simulink model "colorDetectionPID"  (R2022b)
settings: Solver=ode1  StartTime=0.0  StopTime=inf  FixedStep=0.001  RelTol=1e-9
model workspace (MAT data in the model file):
  SL_ROS_VariableLengthArrays_MaxSizes.CommonInfo.ArrayTruncateAction = 'EmitWarning'
  SL_ROS_VariableLengthArrays_MaxSizes.MsgTypeMap = containers.Map
  SL_ROS_VariableLengthArrays_MaxSizes.MsgTypeMap.serialization.keys = {'sensor_msgs/CompressedImage'}
  SL_ROS_VariableLengthArrays_MaxSizes.MsgTypeMap.serialization.values{1}(1).PropertyName = 'Data'
  SL_ROS_VariableLengthArrays_MaxSizes.MsgTypeMap.serialization.values{1}(1).DataType = 'uint8'
  SL_ROS_VariableLengthArrays_MaxSizes.MsgTypeMap.serialization.values{1}(1).MaxLength = 300000
  SL_ROS_VariableLengthArrays_MaxSizes.MsgTypeMap.serialization.values{1}(2).PropertyName = 'Format'
  SL_ROS_VariableLengthArrays_MaxSizes.MsgTypeMap.serialization.values{1}(2).DataType = 'uint8'
  SL_ROS_VariableLengthArrays_MaxSizes.MsgTypeMap.serialization.values{1}(2).MaxLength = 128
  SL_ROS_VariableLengthArrays_MaxSizes.MsgTypeMap.serialization.uniformity = 0
  SL_ROS_VariableLengthArrays_MaxSizes.MsgTypeMap.serialization.keyType = 'char'
  SL_ROS_VariableLengthArrays_MaxSizes.MsgTypeMap.serialization.valueType = 'any'
undefined symbols (not defined in the file): gray, VelLeft, VelRight
libraries: robotlib x11, slpidlib x5, simulink_extras x2, visionsinks x1
settings Model: Creator=domen  LastModifiedBy=gaetano
settings OptimizationCC: EnhancedBackFolding=on  PassReuseOutputArgsAs=Individual arguments  ZeroExternalMemoryAtStartup=off  ZeroInternalMemoryAtStartup=off  MaxStackSize=64  OptimizeBlockOrder=speed  DifferentSizesBufferReuse=on  OptimizationCustomize=off  EfficientTunableParamExpr=on
settings DebuggingCC: ParameterTunabilityLossMsg=error
settings HardwareCC: ProdBitPerPointer=32  ProdBitPerSizeT=32  ProdBitPerPtrDiffT=32  ProdLargestAtomicFloat=None  ProdIntDivRoundTo=Undefined  ProdEndianess=Unspecified  ProdWordSize=32  ProdHWDeviceType=Generic->Unspecified (assume 32-bit Generic)  UseEmbeddedCoderFeatures=off
settings RTWCC: Description=Embedded Coder  SystemTargetFile=ert.tlc  HardwareBoard=Robot Operating System (ROS)  TLCOptions="-aInlineSetEventsForThisBaseRateFcn=TLC_FALSE -aSuppressMultiTaskScheduler=TLC_FALSE  -aRateBasedStepFcn=0"  TemplateMakefile=ert_default_tmf  Toolchain=Catkin  TargetLang=C++
settings CodeAppCC: ForceParamTrailComments=on  IgnoreCustomStorageClasses=off  OperatorAnnotations=on  SimulinkDataObjDesc=on  SFDataObjDesc=on  InsertBlockDesc=on
settings ERTTargetCC: SupportNonInlinedSFcns=on

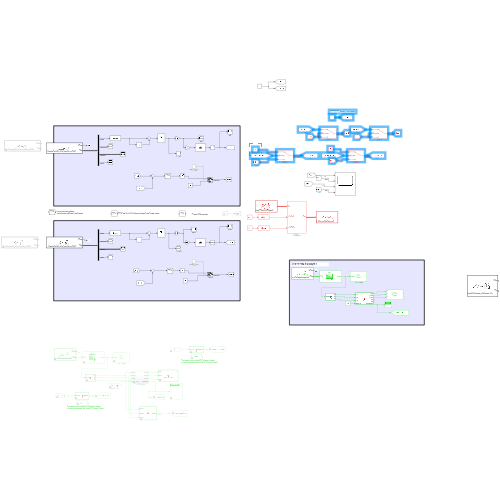
[thumbnail: Simulink's stored preview of the top-level diagram]
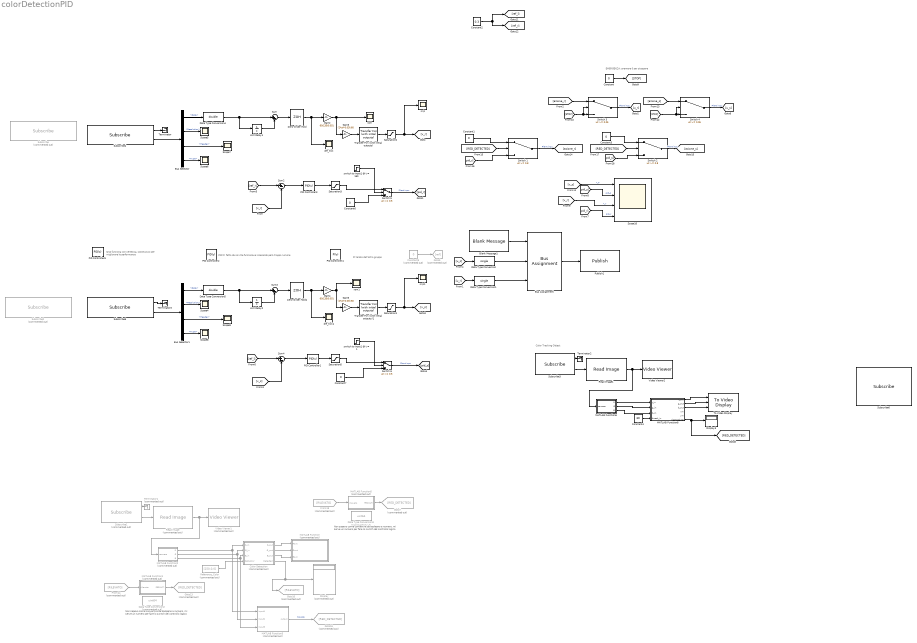
== system colorDetectionPID ==
  note: Color Tracking Object
  note: Non sapevo come convertire da booleano a numero,
      | mi serve un numero per fare lo switch del controllo logico
  note: EMERGENZA: premere 0 per stoppare
  note: 6/12 funziona con certezza,
      |  sostituisco per migliorare le performance
  note: PID(z) fatto da noi che funzionava inserendo però troppo rumore
  note: PI tarato dall'altro gruppo
  note: Non sapevo come convertire da booleano a numero,
      | mi serve un numero per fare lo switch del controllo logico
  Blank Message1 : robotlib/Blank Message  messageClass=Message  entityType=duckietown_msgs/WheelsCmdStamped  messageType=duckietown_msgs/WheelsCmdStamped  SampleTime=-1  legacyBusStruct=off
      settings: LibrarySourceBlock=roslib/ROS/Blank Message
  Bus Assignment : BusAssignment  AssignedSignals=VelLeft,VelRight
  Bus Selector : BusSelector  OutputSignals=Data,Resolution,Header,Type
  Bus Selector1 : BusSelector  OutputSignals=Data,Resolution,Header,Type
  Color Detection : Subsystem  Commented=on
  Constant{,1,3,6..7} (5 alike) : Constant  Value=0
  Constant2 : Constant  Value=0.3
  Constant4 : Constant  Value=30
  Constant5 : Constant  Commented=on  Value=0
  Data Type Conversion : DataTypeConversion  OutDataTypeStr=single  SaturateOnIntegerOverflow=off  RndMeth=Floor
  Data Type Conversion1 : DataTypeConversion  OutDataTypeStr=single  SaturateOnIntegerOverflow=off  RndMeth=Floor
  Data Type Conversion2 : DataTypeConversion  Commented=on  OutMin=[0]  OutMax=[1]  OutDataTypeStr=uint64  SaturateOnIntegerOverflow=off  RndMeth=Floor
  Data Type Conversion3 : DataTypeConversion  Commented=on  OutMin=[0]  OutMax=[1]  OutDataTypeStr=uint64  SaturateOnIntegerOverflow=off  RndMeth=Floor
  Data Type Conversion4 : DataTypeConversion  OutDataTypeStr=double  SaturateOnIntegerOverflow=off  RndMeth=Floor
  Data Type Conversion5 : DataTypeConversion  OutDataTypeStr=double  SaturateOnIntegerOverflow=off  RndMeth=Floor
  Display : Display  Commented=on
  Display3 : Display
  From14 : From  Commented=on  GotoTag=RILEVATO
  From19 : From  Commented=on  GotoTag=RILEVATO
  Gain2 : Gain  Gain=60/135/0.001
  Gain3 : Gain  Gain=(2*pi*0.03)/60
  Gain4 : Gain  Gain=60/135/0.001
  Gain5 : Gain  Gain=(2*pi*0.03)/60
  Goto10 : Goto  Commented=on  GotoTag=RILEVATO
  Goto13 : Goto  Commented=on  GotoTag=RED_DETECTED
  Goto16 : Goto  Commented=on  GotoTag=RED_DETECTED
  Goto5 : Goto  Commented=on  GotoTag=ref
  Goto7 : Goto  Commented=on  GotoTag=RED_DETECTED
  MATLAB Function : MATLAB Function  Commented=on  TreatAsAtomicUnit=on
  MATLAB Function1 : MATLAB Function  Commented=on  TreatAsAtomicUnit=on
  MATLAB Function2 : MATLAB Function  Commented=on  TreatAsAtomicUnit=on
  MATLAB Function3 : MATLAB Function  Commented=on  TreatAsAtomicUnit=on
  MATLAB Function5 : MATLAB Function  Commented=on  TreatAsAtomicUnit=on
  MATLAB Function6 : MATLAB Function  TreatAsAtomicUnit=on
  MATLAB Function8 : MATLAB Function  TreatAsAtomicUnit=on
  PID Controller1 : slpidlib/PID Controller  Controller=PID  Form=Parallel  TimeDomain=Continuous-time  UseExternalTs=off  SampleTime=-1  IntegratorMethod=Forward Euler  FilterMethod=Forward Euler  ControllerParametersSource=internal  P=1.339  I=1.386  UseKiTs=off  D=0.111  N=2.50192573013059  UseFilter=on  TunerSelectOption=Transfer Function Based (PID Tuner App)  InitialConditionSource=internal  InitialConditionForIntegrator=0  InitialConditionForFilter=0  DifferentiatorICPrevScaledInput=0  ExternalReset=none  TrackingMode=off  Kt=1  LimitOutput=off  SatLimitsSource=internal  UpperSaturationLimit=inf  LowerSaturationLimit=-inf  LinearizeAsGain=on  AntiWindupMode=none  Kb=1  LimitIntegrator=off  UpperIntegratorSaturationLimit=inf  LowerIntegratorSaturationLimit=-inf  POutMin=[]  POutMax=[]  IOutMin=[]  IOutMax=[]  DOutMin=[]  DOutMax=[]  NOutMin=[]  NOutMax=[]  SumOutMin=[]  SumOutMax=[]  SaturationOutMin=[]  SaturationOutMax=[]  PParamMin=[]  PParamMax=[]  IParamMin=[]  IParamMax=[]  DParamMin=[]  DParamMax=[]  NParamMin=[]  NParamMax=[]  KbParamMin=[]  KbParamMax=[]  KtParamMin=[]  KtParamMax=[]  KbOutMin=[]  KbOutMax=[]  KtOutMin=[]  KtOutMax=[]  IntegratorOutMin=[]  IntegratorOutMax=[]  FilterOutMin=[]  FilterOutMax=[]  SumI1OutMin=[]  SumI1OutMax=[]  SumI2OutMin=[]  SumI2OutMax=[]  SumI3OutMin=[]  SumI3OutMax=[]  SumI4OutMin=[]  SumI4OutMax=[]  SumDOutMin=[]  SumDOutMax=[]  DifferentiatorOutMin=[]  DifferentiatorOutMax=[]  FilterDiffOutCoefMin=[]  FilterDiffOutCoefMax=[]  ReciprocalOutMin=[]  ReciprocalOutMax=[]  SumDenOutMin=[]  SumDenOutMax=[]  SumNumOutMin=[]  SumNumOutMax=[]  DivideOutMin=[]  DivideOutMax=[]  UdiffTsProdOutMin=[]  UdiffTsProdOutMax=[]  NTsProdOutMin=[]  NTsProdOutMax=[]  UintegralTsProdOutMin=[]  UintegralTsProdOutMax=[]  UngainTsProdOutMin=[]  UngainTsProdOutMax=[]  ClampingZeroOutDataTypeStr=Inherit: Inherit via back propagation  ClampingZeroOutMin=[]  ClampingZeroOutMax=[]  FilterDenConstantOutDataTypeStr=Inherit: Inherit via back propagation  FilterDenConstantOutMin=[]  FilterDenConstantOutMax=[]  PCopyOutDataTypeStr=Inherit: Inherit via back propagation  PCopyOutMin=[]  PCopyOutMax=[]  NCopyOutDataTypeStr=Inherit: Inherit via back propagation  NCopyOutMin=[]  NCopyOutMax=[]  IntegratorContinuousStateAttributes=''  IntegratorStateMustResolveToSignalObject=off  IntegratorRTWStateStorageClass=Auto  FilterContinuousStateAttributes=''  FilterStateMustResolveToSignalObject=off  FilterRTWStateStorageClass=Auto  ParallelPVariant=InternalParameters  IdealPVariant=Disabled  IVariant=InternalParameters  DVariant=InternalParameters  IntegratorVariant=Continuous  SatVariant=Disabled  AWVariant=Passthrough  PCopyVariant=Disabled  TRVariant=Disabled  FdbkBlocksVariant=Forward  IdealPFdbkVariant=Disabled  SatFdbkVariant=Disabled  DerivativeFilterVariant=ContFilter  NVariant=InternalParameters  NCopyVariant=Disabled  FilterICVariant=InternalICsFilter  IntegratorICVariant=InternalICs  ExternalResetVariant=Disabled  TRSumVariant=Passthrough  SumFdbkVariant=Disabled  SumVariant=Sum_PID  TsampFilterVariant=InternalTs  TsampNgainVariant=Passthrough  TsampIntegralVariant=Passthrough  ExternalSaturationOutDataTypeStr=Inherit: Same as second input
  PID Controller2 : slpidlib/PID Controller  Controller=PID  Form=Parallel  TimeDomain=Discrete-time  UseExternalTs=off  SampleTime=-1  IntegratorMethod=Forward Euler  FilterMethod=Forward Euler  ControllerParametersSource=internal  P=1.9258578338098  I=1.64428587710628  UseKiTs=off  D=0.231536267148539  N=3.35803573669718  UseFilter=on  TunerSelectOption=Transfer Function Based (PID Tuner App)  InitialConditionSource=internal  InitialConditionForIntegrator=0  InitialConditionForFilter=0  DifferentiatorICPrevScaledInput=0  ExternalReset=none  TrackingMode=off  Kt=1  LimitOutput=off  SatLimitsSource=internal  UpperSaturationLimit=inf  LowerSaturationLimit=-inf  LinearizeAsGain=on  AntiWindupMode=none  Kb=1  LimitIntegrator=off  UpperIntegratorSaturationLimit=inf  LowerIntegratorSaturationLimit=-inf  POutMin=[]  POutMax=[]  IOutMin=[]  IOutMax=[]  DOutMin=[]  DOutMax=[]  NOutMin=[]  NOutMax=[]  SumOutMin=[]  SumOutMax=[]  SaturationOutMin=[]  SaturationOutMax=[]  PParamMin=[]  PParamMax=[]  IParamMin=[]  IParamMax=[]  DParamMin=[]  DParamMax=[]  NParamMin=[]  NParamMax=[]  KbParamMin=[]  KbParamMax=[]  KtParamMin=[]  KtParamMax=[]  KbOutMin=[]  KbOutMax=[]  KtOutMin=[]  KtOutMax=[]  IntegratorOutMin=[]  IntegratorOutMax=[]  FilterOutMin=[]  FilterOutMax=[]  SumI1OutMin=[]  SumI1OutMax=[]  SumI2OutMin=[]  SumI2OutMax=[]  SumI3OutMin=[]  SumI3OutMax=[]  SumI4OutMin=[]  SumI4OutMax=[]  SumDOutMin=[]  SumDOutMax=[]  DifferentiatorOutMin=[]  DifferentiatorOutMax=[]  FilterDiffOutCoefMin=[]  FilterDiffOutCoefMax=[]  ReciprocalOutMin=[]  ReciprocalOutMax=[]  SumDenOutMin=[]  SumDenOutMax=[]  SumNumOutMin=[]  SumNumOutMax=[]  DivideOutMin=[]  DivideOutMax=[]  UdiffTsProdOutMin=[]  UdiffTsProdOutMax=[]  NTsProdOutMin=[]  NTsProdOutMax=[]  UintegralTsProdOutMin=[]  UintegralTsProdOutMax=[]  UngainTsProdOutMin=[]  UngainTsProdOutMax=[]  ClampingZeroOutDataTypeStr=Inherit: Inherit via back propagation  ClampingZeroOutMin=[]  ClampingZeroOutMax=[]  FilterDenConstantOutDataTypeStr=Inherit: Inherit via back propagation  FilterDenConstantOutMin=[]  FilterDenConstantOutMax=[]  PCopyOutDataTypeStr=Inherit: Inherit via back propagation  PCopyOutMin=[]  PCopyOutMax=[]  NCopyOutDataTypeStr=Inherit: Inherit via back propagation  NCopyOutMin=[]  NCopyOutMax=[]  IntegratorContinuousStateAttributes=''  IntegratorStateMustResolveToSignalObject=off  IntegratorRTWStateStorageClass=Auto  FilterContinuousStateAttributes=''  FilterStateMustResolveToSignalObject=off  FilterRTWStateStorageClass=Auto  ParallelPVariant=InternalParameters  IdealPVariant=Disabled  IVariant=InternalParameters  DVariant=InternalParameters  IntegratorVariant=Discrete  SatVariant=Disabled  AWVariant=Passthrough  PCopyVariant=Disabled  TRVariant=Disabled  FdbkBlocksVariant=Forward  IdealPFdbkVariant=Disabled  SatFdbkVariant=Disabled  DerivativeFilterVariant=ForwardEulerFilter  NVariant=InternalParameters  NCopyVariant=Disabled  FilterICVariant=InternalICsFilter  IntegratorICVariant=InternalICs  ExternalResetVariant=Disabled  TRSumVariant=Passthrough  SumFdbkVariant=Disabled  SumVariant=Sum_PID  TsampFilterVariant=InternalTs  TsampNgainVariant=Passthrough  TsampIntegralVariant=Passthrough  ExternalSaturationOutDataTypeStr=Inherit: Same as second input
  PID Controller3 : slpidlib/PID Controller  Controller=PID  Form=Parallel  TimeDomain=Continuous-time  UseExternalTs=off  SampleTime=-1  IntegratorMethod=Forward Euler  FilterMethod=Forward Euler  ControllerParametersSource=internal  P=1.339  I=1.386  UseKiTs=off  D=0.111  N=2.50192573013059  UseFilter=on  TunerSelectOption=Transfer Function Based (PID Tuner App)  InitialConditionSource=internal  InitialConditionForIntegrator=0  InitialConditionForFilter=0  DifferentiatorICPrevScaledInput=0  ExternalReset=none  TrackingMode=off  Kt=1  LimitOutput=off  SatLimitsSource=internal  UpperSaturationLimit=inf  LowerSaturationLimit=-inf  LinearizeAsGain=on  AntiWindupMode=none  Kb=1  LimitIntegrator=off  UpperIntegratorSaturationLimit=inf  LowerIntegratorSaturationLimit=-inf  POutMin=[]  POutMax=[]  IOutMin=[]  IOutMax=[]  DOutMin=[]  DOutMax=[]  NOutMin=[]  NOutMax=[]  SumOutMin=[]  SumOutMax=[]  SaturationOutMin=[]  SaturationOutMax=[]  PParamMin=[]  PParamMax=[]  IParamMin=[]  IParamMax=[]  DParamMin=[]  DParamMax=[]  NParamMin=[]  NParamMax=[]  KbParamMin=[]  KbParamMax=[]  KtParamMin=[]  KtParamMax=[]  KbOutMin=[]  KbOutMax=[]  KtOutMin=[]  KtOutMax=[]  IntegratorOutMin=[]  IntegratorOutMax=[]  FilterOutMin=[]  FilterOutMax=[]  SumI1OutMin=[]  SumI1OutMax=[]  SumI2OutMin=[]  SumI2OutMax=[]  SumI3OutMin=[]  SumI3OutMax=[]  SumI4OutMin=[]  SumI4OutMax=[]  SumDOutMin=[]  SumDOutMax=[]  DifferentiatorOutMin=[]  DifferentiatorOutMax=[]  FilterDiffOutCoefMin=[]  FilterDiffOutCoefMax=[]  ReciprocalOutMin=[]  ReciprocalOutMax=[]  SumDenOutMin=[]  SumDenOutMax=[]  SumNumOutMin=[]  SumNumOutMax=[]  DivideOutMin=[]  DivideOutMax=[]  UdiffTsProdOutMin=[]  UdiffTsProdOutMax=[]  NTsProdOutMin=[]  NTsProdOutMax=[]  UintegralTsProdOutMin=[]  UintegralTsProdOutMax=[]  UngainTsProdOutMin=[]  UngainTsProdOutMax=[]  ClampingZeroOutDataTypeStr=Inherit: Inherit via back propagation  ClampingZeroOutMin=[]  ClampingZeroOutMax=[]  FilterDenConstantOutDataTypeStr=Inherit: Inherit via back propagation  FilterDenConstantOutMin=[]  FilterDenConstantOutMax=[]  PCopyOutDataTypeStr=Inherit: Inherit via back propagation  PCopyOutMin=[]  PCopyOutMax=[]  NCopyOutDataTypeStr=Inherit: Inherit via back propagation  NCopyOutMin=[]  NCopyOutMax=[]  IntegratorContinuousStateAttributes=''  IntegratorStateMustResolveToSignalObject=off  IntegratorRTWStateStorageClass=Auto  FilterContinuousStateAttributes=''  FilterStateMustResolveToSignalObject=off  FilterRTWStateStorageClass=Auto  ParallelPVariant=InternalParameters  IdealPVariant=Disabled  IVariant=InternalParameters  DVariant=InternalParameters  IntegratorVariant=Continuous  SatVariant=Disabled  AWVariant=Passthrough  PCopyVariant=Disabled  TRVariant=Disabled  FdbkBlocksVariant=Forward  IdealPFdbkVariant=Disabled  SatFdbkVariant=Disabled  DerivativeFilterVariant=ContFilter  NVariant=InternalParameters  NCopyVariant=Disabled  FilterICVariant=InternalICsFilter  IntegratorICVariant=InternalICs  ExternalResetVariant=Disabled  TRSumVariant=Passthrough  SumFdbkVariant=Disabled  SumVariant=Sum_PID  TsampFilterVariant=InternalTs  TsampNgainVariant=Passthrough  TsampIntegralVariant=Passthrough  ExternalSaturationOutDataTypeStr=Inherit: Same as second input
  PID Controller4 : slpidlib/PID Controller  Controller=PI  Form=Parallel  TimeDomain=Continuous-time  UseExternalTs=off  SampleTime=-1  IntegratorMethod=Forward Euler  FilterMethod=Forward Euler  ControllerParametersSource=internal  P=1  I=0.15  UseKiTs=off  D=0  N=100  UseFilter=on  TunerSelectOption=Transfer Function Based (PID Tuner App)  InitialConditionSource=internal  InitialConditionForIntegrator=0  InitialConditionForFilter=0  DifferentiatorICPrevScaledInput=0  ExternalReset=none  TrackingMode=off  Kt=1  LimitOutput=off  SatLimitsSource=internal  UpperSaturationLimit=inf  LowerSaturationLimit=-inf  LinearizeAsGain=on  AntiWindupMode=none  Kb=1  LimitIntegrator=off  UpperIntegratorSaturationLimit=inf  LowerIntegratorSaturationLimit=-inf  POutMin=[]  POutMax=[]  IOutMin=[]  IOutMax=[]  DOutMin=[]  DOutMax=[]  NOutMin=[]  NOutMax=[]  SumOutMin=[]  SumOutMax=[]  SaturationOutMin=[]  SaturationOutMax=[]  PParamMin=[]  PParamMax=[]  IParamMin=[]  IParamMax=[]  DParamMin=[]  DParamMax=[]  NParamMin=[]  NParamMax=[]  KbParamMin=[]  KbParamMax=[]  KtParamMin=[]  KtParamMax=[]  KbOutMin=[]  KbOutMax=[]  KtOutMin=[]  KtOutMax=[]  IntegratorOutMin=[]  IntegratorOutMax=[]  FilterOutMin=[]  FilterOutMax=[]  SumI1OutMin=[]  SumI1OutMax=[]  SumI2OutMin=[]  SumI2OutMax=[]  SumI3OutMin=[]  SumI3OutMax=[]  SumI4OutMin=[]  SumI4OutMax=[]  SumDOutMin=[]  SumDOutMax=[]  DifferentiatorOutMin=[]  DifferentiatorOutMax=[]  FilterDiffOutCoefMin=[]  FilterDiffOutCoefMax=[]  ReciprocalOutMin=[]  ReciprocalOutMax=[]  SumDenOutMin=[]  SumDenOutMax=[]  SumNumOutMin=[]  SumNumOutMax=[]  DivideOutMin=[]  DivideOutMax=[]  UdiffTsProdOutMin=[]  UdiffTsProdOutMax=[]  NTsProdOutMin=[]  NTsProdOutMax=[]  UintegralTsProdOutMin=[]  UintegralTsProdOutMax=[]  UngainTsProdOutMin=[]  UngainTsProdOutMax=[]  ClampingZeroOutDataTypeStr=Inherit: Inherit via back propagation  ClampingZeroOutMin=[]  ClampingZeroOutMax=[]  FilterDenConstantOutDataTypeStr=Inherit: Inherit via back propagation  FilterDenConstantOutMin=[]  FilterDenConstantOutMax=[]  PCopyOutDataTypeStr=Inherit: Inherit via back propagation  PCopyOutMin=[]  PCopyOutMax=[]  NCopyOutDataTypeStr=Inherit: Inherit via back propagation  NCopyOutMin=[]  NCopyOutMax=[]  IntegratorContinuousStateAttributes=''  IntegratorStateMustResolveToSignalObject=off  IntegratorRTWStateStorageClass=Auto  FilterContinuousStateAttributes=''  FilterStateMustResolveToSignalObject=off  FilterRTWStateStorageClass=Auto  ParallelPVariant=InternalParameters  IdealPVariant=Disabled  IVariant=InternalParameters  DVariant=Disabled  IntegratorVariant=Continuous  SatVariant=Disabled  AWVariant=Passthrough  PCopyVariant=Disabled  TRVariant=Disabled  FdbkBlocksVariant=Forward  IdealPFdbkVariant=Disabled  SatFdbkVariant=Disabled  DerivativeFilterVariant=Disabled  NVariant=Disabled  NCopyVariant=Disabled_SignalSpec  FilterICVariant=Disabled  IntegratorICVariant=InternalICs  ExternalResetVariant=Disabled  TRSumVariant=Passthrough  SumFdbkVariant=Disabled  SumVariant=Sum_PI  TsampFilterVariant=InternalTs  TsampNgainVariant=Passthrough  TsampIntegralVariant=Passthrough  ExternalSaturationOutDataTypeStr=Inherit: Same as second input
  PID Controller6 : slpidlib/PID Controller  Controller=PID  Form=Parallel  TimeDomain=Continuous-time  UseExternalTs=off  SampleTime=-1  IntegratorMethod=Forward Euler  FilterMethod=Forward Euler  ControllerParametersSource=internal  P=1.9500021729767  I=2.64652436503106  UseKiTs=off  D=0.143645278367384  N=3.78681783159113  UseFilter=on  TunerSelectOption=Transfer Function Based (PID Tuner App)  InitialConditionSource=internal  InitialConditionForIntegrator=0  InitialConditionForFilter=0  DifferentiatorICPrevScaledInput=0  ExternalReset=none  TrackingMode=off  Kt=1  LimitOutput=off  SatLimitsSource=internal  UpperSaturationLimit=inf  LowerSaturationLimit=-inf  LinearizeAsGain=on  AntiWindupMode=none  Kb=1  LimitIntegrator=off  UpperIntegratorSaturationLimit=inf  LowerIntegratorSaturationLimit=-inf  POutMin=[]  POutMax=[]  IOutMin=[]  IOutMax=[]  DOutMin=[]  DOutMax=[]  NOutMin=[]  NOutMax=[]  SumOutMin=[]  SumOutMax=[]  SaturationOutMin=[]  SaturationOutMax=[]  PParamMin=[]  PParamMax=[]  IParamMin=[]  IParamMax=[]  DParamMin=[]  DParamMax=[]  NParamMin=[]  NParamMax=[]  KbParamMin=[]  KbParamMax=[]  KtParamMin=[]  KtParamMax=[]  KbOutMin=[]  KbOutMax=[]  KtOutMin=[]  KtOutMax=[]  IntegratorOutMin=[]  IntegratorOutMax=[]  FilterOutMin=[]  FilterOutMax=[]  SumI1OutMin=[]  SumI1OutMax=[]  SumI2OutMin=[]  SumI2OutMax=[]  SumI3OutMin=[]  SumI3OutMax=[]  SumI4OutMin=[]  SumI4OutMax=[]  SumDOutMin=[]  SumDOutMax=[]  DifferentiatorOutMin=[]  DifferentiatorOutMax=[]  FilterDiffOutCoefMin=[]  FilterDiffOutCoefMax=[]  ReciprocalOutMin=[]  ReciprocalOutMax=[]  SumDenOutMin=[]  SumDenOutMax=[]  SumNumOutMin=[]  SumNumOutMax=[]  DivideOutMin=[]  DivideOutMax=[]  UdiffTsProdOutMin=[]  UdiffTsProdOutMax=[]  NTsProdOutMin=[]  NTsProdOutMax=[]  UintegralTsProdOutMin=[]  UintegralTsProdOutMax=[]  UngainTsProdOutMin=[]  UngainTsProdOutMax=[]  ClampingZeroOutDataTypeStr=Inherit: Inherit via back propagation  ClampingZeroOutMin=[]  ClampingZeroOutMax=[]  FilterDenConstantOutDataTypeStr=Inherit: Inherit via back propagation  FilterDenConstantOutMin=[]  FilterDenConstantOutMax=[]  PCopyOutDataTypeStr=Inherit: Inherit via back propagation  PCopyOutMin=[]  PCopyOutMax=[]  NCopyOutDataTypeStr=Inherit: Inherit via back propagation  NCopyOutMin=[]  NCopyOutMax=[]  IntegratorContinuousStateAttributes=''  IntegratorStateMustResolveToSignalObject=off  IntegratorRTWStateStorageClass=Auto  FilterContinuousStateAttributes=''  FilterStateMustResolveToSignalObject=off  FilterRTWStateStorageClass=Auto  ParallelPVariant=InternalParameters  IdealPVariant=Disabled  IVariant=InternalParameters  DVariant=InternalParameters  IntegratorVariant=Continuous  SatVariant=Disabled  AWVariant=Passthrough  PCopyVariant=Disabled  TRVariant=Disabled  FdbkBlocksVariant=Forward  IdealPFdbkVariant=Disabled  SatFdbkVariant=Disabled  DerivativeFilterVariant=ContFilter  NVariant=InternalParameters  NCopyVariant=Disabled  FilterICVariant=InternalICsFilter  IntegratorICVariant=InternalICs  ExternalResetVariant=Disabled  TRSumVariant=Passthrough  SumFdbkVariant=Disabled  SumVariant=Sum_PID  TsampFilterVariant=InternalTs  TsampNgainVariant=Passthrough  TsampIntegralVariant=Passthrough  ExternalSaturationOutDataTypeStr=Inherit: Same as second input
  Publish1 : robotlib/Publish  topicSource=Select from ROS network  topic=/vic9osimhen/wheels_driver_node/wheels_cmd  messageType=duckietown_msgs/WheelsCmdStamped  legacyBusStruct=off  messageQueueLength=1
      settings: LibrarySourceBlock=roslib/ROS/Publish
  Read Image : robotlib/Read Image  Commented=on  MaximumImageSize=[ 2000, 2000 ]  ImageEncoding=rgb8  ShowAlphaOutput=off  ShowErrorCodeOutput=off  VariableSizeOutputs=off
      settings: LibrarySourceBlock=roslib/ROS/Read Image
  Read Image1 : robotlib/Read Image  MaximumImageSize=[480, 640 ]  ImageEncoding=rgb8  ShowAlphaOutput=off  ShowErrorCodeOutput=off  VariableSizeOutputs=off
      settings: LibrarySourceBlock=roslib/ROS/Read Image
  Reference_Color : Constant  Commented=on  Value=[150,0,0]  OutDataTypeStr=uint8
  Saturation{1..3,5} (4 alike) : Saturate  UpperLimit=0.95  LowerLimit=-0.95
  Scope10 : Scope  NumInputPorts=4
  Scope{4..9} (6 alike) : Scope
  Subscribe : robotlib/Subscribe  Commented=on  topicSource=Select from ROS network  topic=/diegodemme4/right_wheel_encoder_node/tick  messageType=duckietown_msgs/WheelEncoderStamped  SampleTime=-1  legacyBusStruct=off  messageQueueLength=1
      settings: LibrarySourceBlock=roslib/ROS/Subscribe
  Subscribe1 : robotlib/Subscribe  Commented=on  topicSource=Select from ROS network  topic=/diegodemme4/camera_node/image/compressed  messageType=sensor_msgs/CompressedImage  SampleTime=0.1  legacyBusStruct=off  messageQueueLength=1
      settings: LibrarySourceBlock=roslib/ROS/Subscribe
  Subscribe2 : robotlib/Subscribe  Commented=on  topicSource=Select from ROS network  topic=/diegodemme4/left_wheel_encoder_node/tick  messageType=duckietown_msgs/WheelEncoderStamped  SampleTime=-1  legacyBusStruct=off  messageQueueLength=1
      settings: LibrarySourceBlock=roslib/ROS/Subscribe
  Subscribe3 : robotlib/Subscribe  topicSource=Select from ROS network  topic=/vic9osimhen/camera_node/image/compressed  messageType=sensor_msgs/CompressedImage  SampleTime=0.1  legacyBusStruct=off  messageQueueLength=1
      settings: LibrarySourceBlock=roslib/ROS/Subscribe
  Subscribe4 : robotlib/Subscribe  topicSource=Select from ROS network  topic=/vic9osimhen/right_wheel_encoder_node/tick  messageType=duckietown_msgs/WheelEncoderStamped  SampleTime=-1  legacyBusStruct=off  messageQueueLength=1
      settings: LibrarySourceBlock=roslib/ROS/Subscribe
  Subscribe5 : robotlib/Subscribe  topicSource=Select from ROS network  topic=/vic9osimhen/left_wheel_encoder_node/tick  messageType=duckietown_msgs/WheelEncoderStamped  SampleTime=-1  legacyBusStruct=off  messageQueueLength=1
      settings: LibrarySourceBlock=roslib/ROS/Subscribe
  Subscribe6 : robotlib/Subscribe  topicSource=Select from ROS network  topic=/vic9osimhen/camera_node/camera_info  messageType=sensor_msgs/CameraInfo  SampleTime=-1  legacyBusStruct=off  messageQueueLength=1
      settings: LibrarySourceBlock=roslib/ROS/Subscribe
  Sum{,2..4} (4 alike) : Sum  Inputs=|+-
  Switch 1 : Switch  Threshold=0.8  SaturateOnIntegerOverflow=off  InputSameDT=off
  Switch 2 : Switch  Threshold=0.8  SaturateOnIntegerOverflow=off  InputSameDT=off
  Switch 3 : Switch  Threshold=0.05  SaturateOnIntegerOverflow=off  InputSameDT=off
  Switch 4 : Switch  Threshold=0.05  SaturateOnIntegerOverflow=off  InputSameDT=off
  Switch 5 : Switch  Threshold=0.5  SaturateOnIntegerOverflow=off  InputSameDT=off
  Switch 6 : Switch  Threshold=0.5  SaturateOnIntegerOverflow=off  InputSameDT=off
  Terminator : Terminator
  Terminator1 : Terminator  Commented=on
  Terminator2 : Terminator
  Terminator3 : Terminator
  To Video Display : visionsinks/To Video Display  windowSizeMode=Normal  openAtMdlStart=on  fullScreen=off  videoWindowX=1186  videoWindowY=599  saveWindowSize=off  videoWindowWidth=640  videoWindowHeight=480  inputColorFormat=RGB  inputType=Obsolete  imagePorts=Separate color signals  OutputDevice=On-screen video monitor  dataOrg=Column-major  isWindowOpen=off
  Transfer Fcn (with initial outputs) : simulink_extras/Additional Linear/Transfer Fcn (with initial outputs)  N=[1]  D="[1  1]"  Y0=0  U0=0
  Transfer Fcn (with initial outputs)1 : simulink_extras/Additional Linear/Transfer Fcn (with initial outputs)  N=[1]  D="[1  1]"  Y0=0  U0=0
  Unit Delay1 : UnitDelay  SampleTime=-1  HasFrameUpgradeWarning=on
  Unit Delay2 : UnitDelay  SampleTime=-1  HasFrameUpgradeWarning=on
  Video Viewer1 : VideoViewer  Commented=on  colormapValue=gray(256)  FigPos=[609.8 719.6 645.6 521.6]
  Video Viewer2 : VideoViewer  colormapValue=gray(256)  FigPos=[144.2 826 873.6 633]
  Zero-Order Hold : ZeroOrderHold  SampleTime=-1
  Zero-Order Hold1 : ZeroOrderHold  SampleTime=-1
  diff_tick : Scope
  diff_tick1 : Scope
  m/s : Scope
  m/s1 : Scope
  rpm : Scope
  rpm1 : Scope
  switch to input1 @ t = 1 : Step  Time=13  SampleTime=0
  switch to input1 @ t = 150 : Step  Time=13  SampleTime=0
  wires:
  Bus Assignment/1 -> Publish1/1
  Blank Message1/1 -> Bus Assignment/1
  Subscribe4/1 -> Terminator/1
  Subscribe4/2 -> Bus Selector/1
  Data Type Conversion/1 -> Bus Assignment/2
  Data Type Conversion1/1 -> Bus Assignment/3
  [u_s] -> Data Type Conversion/1
  Bus Selector/2 -> Scope5/1  "<Resolution>"
  Bus Selector/3 -> Scope7/1  "<Header>"
  Bus Selector/4 -> Scope6/1  "<Type>"
  Bus Selector/1 -> Data Type Conversion4/1  "<Data>"
  Sum/1 -> Zero-Order Hold/1
  Gain2/1 -> Gain3/1, rpm/1
  Gain3/1 -> Transfer Fcn (with initial outputs)/1
  Zero-Order Hold/1 -> Gain2/1, diff_tick/1
  Unit Delay1/1 -> Sum/2
  Data Type Conversion4/1 -> Unit Delay1/1, Sum/1
  Transfer Fcn (with initial outputs)/1 -> Saturation2/1
  [ref_r] -> Sum2/1
  [v_r] -> Sum2/2
  [u_r] -> Data Type Conversion1/1
  Sum2/1 -> PID Controller3/1
  Subscribe5/1 -> Terminator3/1
  Bus Selector1/1 -> Data Type Conversion5/1  "<Data>"
  Bus Selector1/4 -> Scope8/1  "<Type>"
  Subscribe5/2 -> Bus Selector1/1
  Gain5/1 -> Transfer Fcn (with initial outputs)1/1
  Bus Selector1/3 -> Scope9/1  "<Header>"
  Zero-Order Hold1/1 -> Gain4/1, diff_tick1/1
  Gain4/1 -> Gain5/1, rpm1/1
  Unit Delay2/1 -> Sum3/2
  Data Type Conversion5/1 -> Unit Delay2/1, Sum3/1
  Bus Selector1/2 -> Scope4/1  "<Resolution>"
  Transfer Fcn (with initial outputs)1/1 -> Saturation1/1
  Sum3/1 -> Zero-Order Hold1/1
  [ref_l] -> Sum4/1
  Sum4/1 -> PID Controller1/1
  [v_s] -> Sum4/2
  [pid_s] -> Scope10/2  "pid_s"
  [pid_r] -> Scope10/4  "pid_r"
  [v_r] -> Scope10/3  "v_r"
  [v_s] -> Scope10/1  "v_s"
  Constant5/1 -> Goto5/1
  [STOP] -> Switch 3/2, Switch 3/3
  Switch 3/1 -> [u_r]  "Plant inpu"
  [azione_r] -> Switch 3/1
  [STOP] -> Switch 4/2, Switch 4/3
  [azione_s] -> Switch 4/1
  Switch 4/1 -> [u_s]  "Plant inpu"
  Constant/1 -> [STOP]
  Constant2/1 -> [ref_l], [ref_r]
  Read Image/1 -> MATLAB Function2/1(camera), Video Viewer1/1
  Subscribe1/2 -> Read Image/1
  Subscribe1/1 -> Terminator1/1
  Color Detection/2(G_out) -> MATLAB Function/2(Gout)
  Color Detection/3(B_out) -> MATLAB Function/3(Bout)
  Color Detection/1(R_out) -> MATLAB Function/1(Rout)
  Color Detection/4(Detected) -> Display/1, Goto10/1
  From14/1 -> MATLAB Function1/1(rilevato)
  MATLAB Function1/1(FERMATI) -> Goto13/1
  Reference_Color/1 -> Color Detection/4(Ref_color)
  [RED_DETECTED] -> Switch 1/2
  Switch 1/1 -> [azione_r]  "Plant inpu"
  Switch 2/1 -> [azione_s]  "Plant inpu"
  [RED_DETECTED] -> Switch 2/2
  MATLAB Function2/1(R) -> Color Detection/1(R_in), MATLAB Function3/1(input1)
  MATLAB Function2/2(G) -> Color Detection/2(G_in), MATLAB Function3/2(input2)
  MATLAB Function2/3(B) -> Color Detection/3(B_in), MATLAB Function3/3(input3)
  MATLAB Function3/1(output) -> Goto16/1  "trovato"
  Constant1/1 -> Switch 1/1
  [pid_r] -> Switch 1/3
  Constant3/1 -> Switch 2/1
  [pid_s] -> Switch 2/3
  MATLAB Function8/6(riconosciuto) -> [RED_DETECTED], Display3/1
  Constant4/1 -> MATLAB Function8/4(thresh_in)
  MATLAB Function8/2(g_out) -> To Video Display/2
  MATLAB Function8/1(r_out) -> To Video Display/1
  Read Image1/1 -> MATLAB Function6/1(camera), Video Viewer2/1
  Subscribe3/1 -> Terminator2/1
  MATLAB Function6/2(G) -> MATLAB Function8/2(g_in)
  Subscribe3/2 -> Read Image1/1
  MATLAB Function5/1(FERMATI) -> Goto7/1
  MATLAB Function6/3(B) -> MATLAB Function8/3(b_in)
  MATLAB Function6/1(R) -> MATLAB Function8/1(r_in)
  MATLAB Function8/3(b_out) -> To Video Display/3
  From19/1 -> MATLAB Function5/1(rilevato)
  Switch 5/1 -> [pid_r]  "Plant inpu"
  PID Controller3/1 -> Saturation3/1
  Saturation3/1 -> Switch 5/1
  switch to input1 @ t = 150/1 -> Switch 5/2
  Constant6/1 -> Switch 5/3
  Switch 6/1 -> [pid_s]  "Plant inpu"
  PID Controller1/1 -> Saturation5/1
  Constant7/1 -> Switch 6/3
  Saturation5/1 -> Switch 6/1
  switch to input1 @ t = 1/1 -> Switch 6/2
  Saturation1/1 -> m/s1/1, [v_s]
  Saturation2/1 -> m/s/1, [v_r]

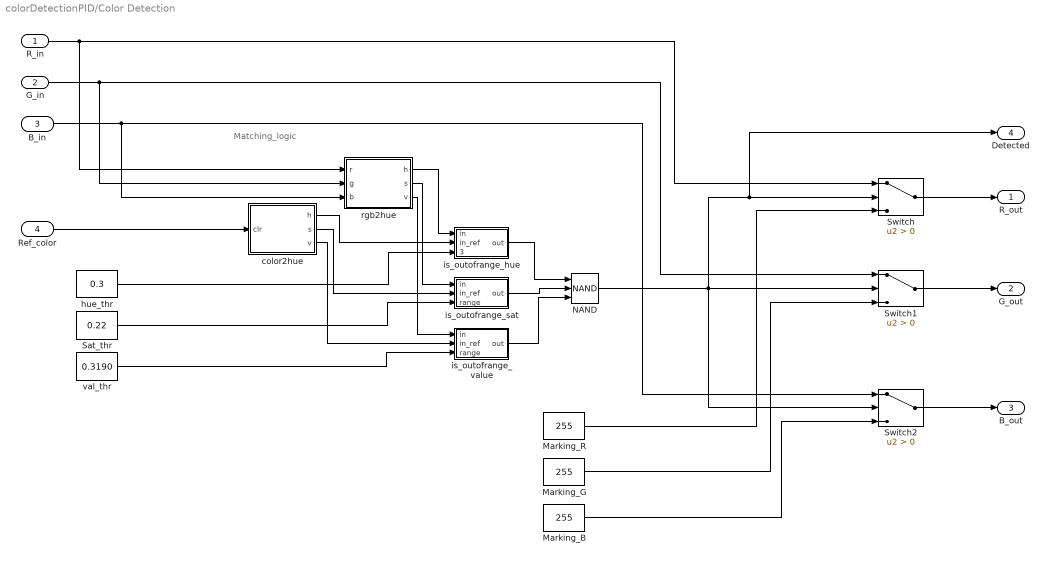
== system colorDetectionPID/Color Detection ==
  note: Matching_logic
  R_in : Inport
  G_in : Inport  Port=2
  B_in : Inport  Port=3
  Ref_color : Inport  Port=4
  Marking_B : Constant  Value=255
  Marking_G : Constant  Value=255
  Marking_R : Constant  Value=255
  NAND : Logic  Operator=NAND  Inputs=3  IconShape=distinctive  AllPortsSameDT=off  OutDataTypeStr=boolean
  Sat_thr : Constant  Value=0.22
  Switch : Switch  Criteria=u2 > Threshold  OutDataTypeStr=uint8  SaturateOnIntegerOverflow=off  InputSameDT=off
  Switch1 : Switch  Criteria=u2 > Threshold  OutDataTypeStr=uint8  SaturateOnIntegerOverflow=off  InputSameDT=off
  Switch2 : Switch  Criteria=u2 > Threshold  OutDataTypeStr=uint8  SaturateOnIntegerOverflow=off  InputSameDT=off
  color2hue : MATLAB Function  TreatAsAtomicUnit=on
  hue_thr : Constant  Value=0.3
  is_outofrange_hue : Subsystem
  "is_outofrange_sat " : Subsystem
  is_outofrange_value : Subsystem
  rgb2hue : MATLAB Function  TreatAsAtomicUnit=on
  val_thr : Constant  Value=0.3190
  R_out : Outport
  G_out : Outport  Port=2
  B_out : Outport  Port=3
  Detected : Outport  Port=4
  wires:
  NAND/1 -> Switch2/2, Switch1/2, Detected/1, Switch/2
  hue_thr/1 -> is_outofrange_hue/3("threshold ")
  is_outofrange_value/1(out) -> NAND/3
  is_outofrange_hue/1(out) -> NAND/1
  Sat_thr/1 -> "is_outofrange_sat "/3("range ")
  val_thr/1 -> is_outofrange_value/3("range ")
  rgb2hue/3(v) -> is_outofrange_value/1(in)
  color2hue/3(v) -> is_outofrange_value/2(in_ref)
  color2hue/1(h) -> is_outofrange_hue/2(in_ref)
  rgb2hue/1(h) -> is_outofrange_hue/1(in)
  Ref_color/1 -> color2hue/1(clr)
  "is_outofrange_sat "/1(out) -> NAND/2
  color2hue/2(s) -> "is_outofrange_sat "/2(in_ref)
  G_in/1 -> Switch1/1, rgb2hue/2(g)
  rgb2hue/2(s) -> "is_outofrange_sat "/1(in)
  B_in/1 -> Switch2/1, rgb2hue/3(b)
  R_in/1 -> rgb2hue/1(r), Switch/1
  Marking_R/1 -> Switch/3
  Switch/1 -> R_out/1
  Switch1/1 -> G_out/1
  Switch2/1 -> B_out/1
  Marking_G/1 -> Switch1/3
  Marking_B/1 -> Switch2/3

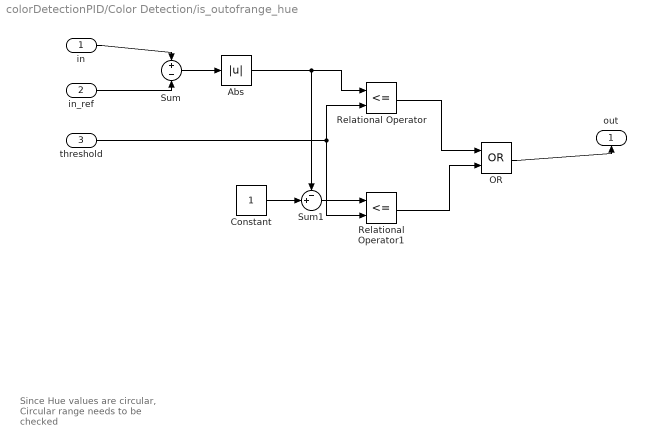
== system colorDetectionPID/Color Detection/is_outofrange_hue ==
  note: Since Hue values are circular, Circular range needs to be checked
  in : Inport
  in_ref : Inport  Port=2
  "threshold " : Inport  Port=3
  Abs : Abs  SaturateOnIntegerOverflow=off
  Constant : Constant
  "OR " : Logic  Operator=OR  AllPortsSameDT=off  OutDataTypeStr=boolean
  Relational Operator : RelationalOperator  Operator=<=  OutDataTypeStr=boolean  InputSameDT=off
  Relational Operator1 : RelationalOperator  Operator=<=  OutDataTypeStr=boolean  InputSameDT=off
  Sum : Sum  Inputs=+|-
  Sum1 : Sum  Inputs=-+|
  out : Outport
  wires:
  in/1 -> Sum/1
  in_ref/1 -> Sum/2
  Sum/1 -> Abs/1
  Abs/1 -> Sum1/1, Relational Operator/1
  "threshold "/1 -> Relational Operator1/2, Relational Operator/2
  Constant/1 -> Sum1/2
  Sum1/1 -> Relational Operator1/1
  Relational Operator/1 -> "OR "/1
  Relational Operator1/1 -> "OR "/2
  "OR "/1 -> out/1

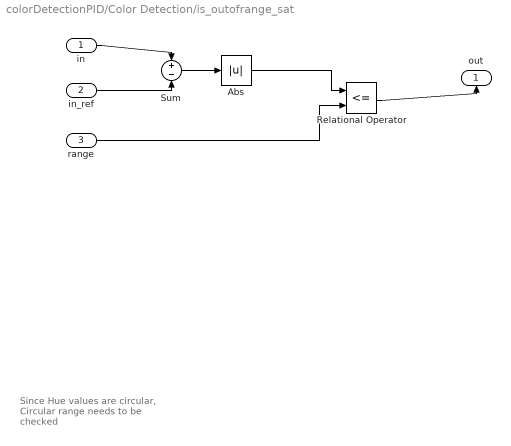
== system colorDetectionPID/Color Detection/is_outofrange_sat  ==
  note: Since Hue values are circular, Circular range needs to be checked
  in : Inport
  in_ref : Inport  Port=2
  "range " : Inport  Port=3
  Abs : Abs  SaturateOnIntegerOverflow=off
  Relational Operator : RelationalOperator  Operator=<=  OutDataTypeStr=boolean  InputSameDT=off
  Sum : Sum  Inputs=+|-
  out : Outport
  wires:
  in/1 -> Sum/1
  in_ref/1 -> Sum/2
  Sum/1 -> Abs/1
  Abs/1 -> Relational Operator/1
  "range "/1 -> Relational Operator/2
  Relational Operator/1 -> out/1

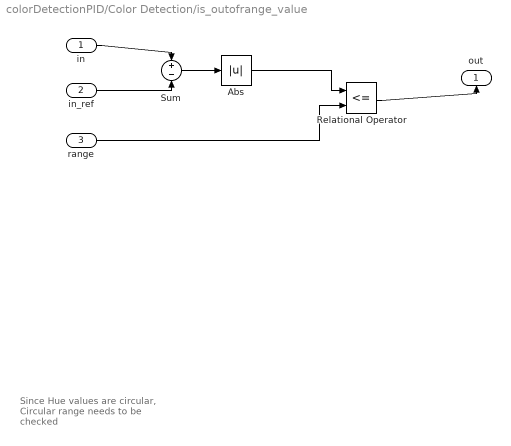
== system colorDetectionPID/Color Detection/is_outofrange_value ==
  note: Since Hue values are circular, Circular range needs to be checked
  in : Inport
  in_ref : Inport  Port=2
  "range " : Inport  Port=3
  Abs : Abs  SaturateOnIntegerOverflow=off
  Relational Operator : RelationalOperator  Operator=<=  OutDataTypeStr=boolean  InputSameDT=off
  Sum : Sum  Inputs=+|-
  out : Outport
  wires:
  in/1 -> Sum/1
  in_ref/1 -> Sum/2
  Sum/1 -> Abs/1
  Abs/1 -> Relational Operator/1
  "range "/1 -> Relational Operator/2
  Relational Operator/1 -> out/1

== matlab function colorDetectionPID/MATLAB Function5 ==
  data: rilevato input; FERMATI output
function FERMATI= fcn(rilevato)

if rilevato==1
    FERMATI=0;
else
    FERMATI=1;
end

== matlab function colorDetectionPID/MATLAB Function6 ==
  data: camera input; R output; G output; B output
function [R,G,B] = fcn(camera)


[R,G,B]=imsplit(camera);

== matlab function colorDetectionPID/MATLAB Function8 ==
  data: r_in input; r_out output; g_in input; b_in input; thresh_in input; g_out output; b_out output; xm output; ym output; riconosciuto output
% function [r_out,g_out,b_out, xm,ym,riconosciuto] = fcn(r_in,g_in,b_in,thresh_in) 
% %#codegen 
% %%Get RGB color 
% r=r_in; 
% g=g_in; 
% b=b_in; 
% thresh=thresh_in; 
% %%calculate green 
% justGreen=g-r/2-b/2; 
% %%threshold the image 
% bw=justGreen>thresh; 
% %%find center 
% [x,y]=find(bw); 
% xm=mean(x); 
% ym=mean(y); 
% %%creat the red dot 
% xx=max(1,xm-5):min(xm+5,size(bw,1)); 
% yy=max(1,ym-5):min(ym+5,size(bw,2)); 
% bwbw=zeros(size(bw),'uint8'); 
% bwbw(uint16(xx),uint16(yy))=255; 
% % Calcola il valore medio della componente verde nella regione
% green_mean = mean(mean(g_in(uint16(xx), uint16(yy))));
%  % Imposta il flag 'riconosciuto' in base al valore medio
% riconosciuto = green_mean > thresh_in;
%     % Modifica l'output RGB in base al flag 'riconosciuto'
%     if riconosciuto
%         r_out = uint8(double(r_in) + double(bwbw));
%         g_out = uint8(double(g_in) - double(bwbw));
%         b_out = uint8(double(b_in) - double(bwbw));
%     else
%         % Se il verde non viene riconosciuto, mantieni l'immagine originale
%         r_out = r_in;
%         g_out = g_in;
%         b_out = b_in;
%     end
% end

function [r_out, g_out, b_out, xm, ym, riconosciuto] = fcn(r_in, g_in, b_in, thresh_in)
    % Get RGB color
    r = r_in;
    g = g_in;
    b = b_in;
    thresh = thresh_in;
 
    % Calcola il canale verde modificato
    justGreen = g - r/2 - b/2;
 
    % Soglia dell'immagine
    bw = justGreen > thresh;
 
    % Applica una condizione aggiuntiva basata sui valori dei canali RGB
    greenCondition = (g > 50) & (r < 100) & (b < 100);
    bw = bw & greenCondition;
 
    % Trova il centro
    [x, y] = find(bw);
    xm = mean(x);
    ym = mean(y);
 
    % Crea il rettangolo rosso
    xx = max(1, xm - 5):min(xm + 5, size(bw, 1));
    yy = max(1, ym - 5):min(ym + 5, size(bw, 2));
    bwbw = zeros(size(bw), 'uint8');
    bwbw(uint16(xx), uint16(yy)) = 255;
 
    % Sovrapposizione dei rettangoli all'immagine originale
    r_out = uint8(double(r_in) + double(bwbw));
    g_out = uint8(double(g_in) - double(bwbw));
    b_out = uint8(double(b_in) - double(bwbw));
 
    % Verifica se il verde è stato riconosciuto
    if any(bw(:))
        riconosciuto = 1;
    else
        riconosciuto = 0;
    end
end

== matlab function colorDetectionPID/Color Detection/color2hue ==
  data: clr input; h output; s output; v output
function [h,s,v] = color2hue(clr)
%#codegen

hsv = rgb2hsv(double(clr')/255.0);
h = hsv(1);
s = hsv(2);
v = hsv(3);

== matlab function colorDetectionPID/Color Detection/rgb2hue ==
  data: r input; h output; g input; b input; s output; v output
function [h,s,v] = rgb2hue(r,g,b)
%#codegen

sz = size(r);
r_re = double(reshape(r,[sz(1)*sz(2),1]))/255.0;
g_re = double(reshape(g,[sz(1)*sz(2),1]))/255.0;
b_re = double(reshape(b,[sz(1)*sz(2),1]))/255.0;
hsv = rgb2hsv([r_re,g_re,b_re]);
h = reshape(hsv(:,1), sz);
s = reshape(hsv(:,2), sz);
v = reshape(hsv(:,3), sz);

== matlab function colorDetectionPID/MATLAB Function ==
  data: Rout input; Gout input; Bout input
function image_display(Rout,Gout,Bout)
% image_display is MatLAB function block created to automatically display
% an RGB channel stream as an image using imshow matlab command
%
% See also 'imshow'
    RGB_out = uint8(ones([size(Rout) 3]));
    RGB_out(:,:,1) = uint8(Rout);
    RGB_out(:,:,2) = uint8(Gout);
    RGB_out(:,:,3) = uint8(Bout);
    
    % Declaration to use 'imshow' with coder.extrinsic
    coder.extrinsic('imshow');  
    persistent hFig; % Figure variable and reusing it for display
    if isempty(hFig)
        hFig = figure('Position',[0 0 1024 768]);
    end
    imshow(RGB_out); % Display image in figure
end

== matlab function colorDetectionPID/MATLAB Function1 ==
  data: rilevato input; FERMATI output
function FERMATI= fcn(rilevato)

if rilevato==1
    FERMATI=0;
else
    FERMATI=1;
end

== matlab function colorDetectionPID/MATLAB Function2 ==
  data: camera input; R output; G output; B output
function [R,G,B] = fcn(camera)


[R,G,B]=imsplit(camera);

== matlab function colorDetectionPID/MATLAB Function3 ==
  data: input1 input; output output; input2 input; input3 input
function output = fcn(input1,input2,input3)

R=input1;
G=input2;
B=input3;

image= uint8(ones([size(R) 3]));
    image(:,:,1) = uint8(R);
    image(:,:,2) = uint8(G);
    image(:,:,3) = uint8(B);



% Converti l'immagine da RGB a HSV
hsvImage = rgb2hsv(image);

% Estrai i canali HSV
hChannel = hsvImage(:,:,1); % Canale tonalità

% Definisci le soglie per il rilevamento del rosso nel canale tonalità
redThreshold = 0.95; % Valori tipici per il rosso, ma potrebbero variare

% Trova i pixel che corrispondono alla tonalità del rosso
redPixels = hChannel > redThreshold;

% Verifica se ci sono pixel rossi nell'immagine
if any(redPixels(:)) % matrice che mette a 1 le posizioni in cui è presente il rosso
    % Se ci sono pixel rossi, imposta la variabile a 1
    output = 1;
else
    % Altrimenti, la variabile rimane 0
    output = 0;
end

end
